simulink model "sgMdl_CAN_FDLoopback"  (R2024b)
settings: Solver=FixedStepAuto  StartTime=0.0  StopTime=inf  RelTol=1e-3  EnableMultiTasking=on
undefined symbols (not defined in the file): CAN, Down, FD, IO602, Pull
libraries: canfdmsglib x7, speedgoatlib_IO602_4 x7, simulink x3, canmsglib x1
Description:
  | CAN - Working with CAN FD
settings Model: ModifiedByFormat=Speedgoat  SimulationMode=external  ExtModeEnableFloating=off  ExtModeTrigDuration=100000  Creator=Speedgoat  LastModifiedBy=Speedgoat
settings SolverCC: ConcurrentTasks=on  AlgebraicLoopSolver=TrustRegion  PositivePriorityOrder=on  AutoInsertRateTranBlk=on  InsertRTBMode=Never (minimum delay)
settings DataIOCC: SaveFormat=StructureWithTime
settings OptimizationCC: BlockReduction=off  OptimizeBlockIOStorage=off  BufferReuse=off  ReuseModelBlockBuffer=off  GlobalBufferReuse=off  ExpressionFolding=off  LocalBlockOutputs=off  OptimizeDataStoreBuffers=off  BusAssignmentInplaceUpdate=off
settings DebuggingCC: InheritedTsInSrcMsg=none  TasksWithSamePriorityMsg=none  ParameterPrecisionLossMsg=none  UnconnectedInputMsg=warning  UnconnectedOutputMsg=warning  UnconnectedLineMsg=warning
settings HardwareCC: ProdBitPerLong=64  ProdLongLongMode=on  ProdHWDeviceType=Intel->x86-64 (Linux 64)
settings ModelReferenceCC: EnableRefExpFcnMdlSchedulingChecks=on
settings SFSimCC: CustomCodeUndefinedFunction=UseInterfaceOnly
settings RTWCC: Description=Speedgoat Real-Time Target Machine  SystemTargetFile=speedgoat.tlc  TemplateMakefile=slrealtime_default_tmf  Toolchain=Simulink Real-Time Toolchain  BuildConfiguration=Faster Runs  TargetLang=C++  GPUComputeCapability=3.5  DLArmComputeVersion=19.05
settings SimulinkRealTimeTargetCC: SubcomponentCodeInterfacePackaging=Reusable function  InstructionSetFMA=off  LogToMDFFile=off  SLRTFileLogMaxRuns=10  UseGCCFastMath=on
settings ConfigComp: CovBoundaryAbsTol=1.0e-5

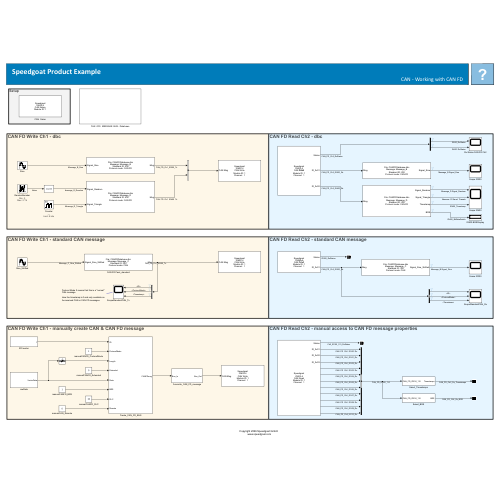
[thumbnail: Simulink's stored preview of the top-level diagram]
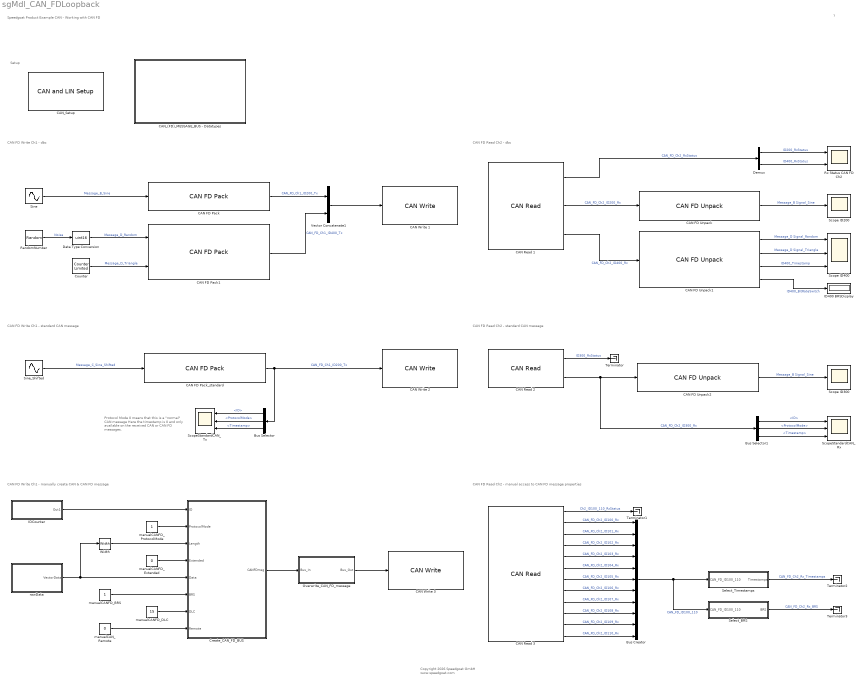
== system sgMdl_CAN_FDLoopback ==
  note: Setup
  note: CAN FD Write Ch1 - dbc
  note: CAN FD Read Ch2 - dbc
  note: CAN FD Write Ch1 - standard CAN message
  note: CAN FD Read Ch2 - standard CAN message
  note: CAN FD Write Ch1 - manually create CAN & CAN FD message
  note: CAN FD Read Ch2 - manual access to CAN FD message properties
  note: Protocol Mode 0 means that this is a "normal" CAN message
      |
      | Here the timestamp is 0 and only available on the received CAN or CAN FD messages.
  note: Speedgoat Product Example
      | CAN - Working with CAN FD
  note: ?
  note: Copyright 2026 Speedgoat GmbH
      |  www.speedgoat.com
  Bus Creator : BusCreator  Inputs=11
  Bus Selector : BusSelector  OutputSignals=ID,ProtocolMode,Timestamp
  Bus Selector1 : BusSelector  OutputSignals=ID,ProtocolMode,Timestamp
  CAN FD Pack : canfdmsglib/CAN FD Pack  CANdbFile=CANFDDatabase.dbc  MsgList=(none)  MsgName=Message_B  ProtocolMode=CAN FD  MsgIDType=Standard (11-bit identifier)  MsgIdentifier=200  CANIDInput=off  MsgLength=8  Remote=off  BRSSwitch=on  ApplyMinMax=off  SignalInfo={'Signal_Sine','0','64','LE','double','Standard','0','1','0','-1.7e+308','1.7e+308'}
      settings: DataFormat=CANdb specified signals
  CAN FD Pack1 : canfdmsglib/CAN FD Pack  CANdbFile=CANFDDatabase.dbc  MsgList=(none)  MsgName=Message_D  ProtocolMode=CAN FD  MsgIDType=Standard (11-bit identifier)  MsgIdentifier=400  CANIDInput=off  MsgLength=3  Remote=off  BRSSwitch=on  ApplyMinMax=off  SignalInfo={'Signal_Random','0','16','LE','unsigned','Standard','0','1','0','0','65535';'Signal_Triangle','16','8','LE','signed','Standard','0','1','0','-128','127'}
      settings: DataFormat=CANdb specified signals
  CAN FD Pack_standard : canfdmsglib/CAN FD Pack  CANdbFile=CANFDDatabase.dbc  MsgList=(none)  MsgName=Message_C  ProtocolMode=CAN  MsgIDType=Standard (11-bit identifier)  MsgIdentifier=300  CANIDInput=off  MsgLength=8  Remote=off  BRSSwitch=off  ApplyMinMax=off  SignalInfo={'Signal_Sine_Shifted','0','64','LE','double','Standard','0','1','0','-1.7e+308','1.7e+308'}
      settings: DataFormat=CANdb specified signals
  CAN FD Unpack : canfdmsglib/CAN FD Unpack  CANdbFile=CANFDDatabase.dbc  MsgList=(none)  MsgName=Message_B  ProtocolMode=CAN FD  MsgIDType=Standard (11-bit identifier)  MsgIdentifier=200  MsgLength=8  SignalInfo={'Signal_Sine','0','64','LE','double','Standard','0','1','0','-1.7e+308','1.7e+308'}  IDPort=off  TimestampPort=off  ErrorPort=off  RemotePort=off  LengthPort=off  StatusPort=off  BRSPort=off  ESIPort=off  DLCPort=off  ApplyMinMax=off
      settings: DataFormat=CANdb specified signals
  CAN FD Unpack1 : canfdmsglib/CAN FD Unpack  CANdbFile=CANFDDatabase.dbc  MsgList=(none)  MsgName=Message_D  ProtocolMode=CAN FD  MsgIDType=Standard (11-bit identifier)  MsgIdentifier=400  MsgLength=3  SignalInfo={'Signal_Random','0','16','LE','unsigned','Standard','0','1','0','0','65535';'Signal_Triangle','16','8','LE','signed','Standard','0','1','0','-128','127'}  IDPort=off  TimestampPort=on  ErrorPort=off  RemotePort=off  LengthPort=off  StatusPort=off  BRSPort=on  ESIPort=off  DLCPort=off  ApplyMinMax=off
      settings: DataFormat=CANdb specified signals
  CAN FD Unpack2 : canfdmsglib/CAN FD Unpack  CANdbFile=CANFDDatabase.dbc  MsgList=(none)  MsgName=Message_C  ProtocolMode=CAN  MsgIDType=Standard (11-bit identifier)  MsgIdentifier=300  MsgLength=8  SignalInfo={'Signal_Sine_Shifted','0','64','LE','double','Standard','0','1','0','-1.7e+308','1.7e+308'}  IDPort=off  TimestampPort=off  ErrorPort=off  RemotePort=off  LengthPort=off  StatusPort=off  BRSPort=off  ESIPort=off  DLCPort=off  ApplyMinMax=off
      settings: DataFormat=CANdb specified signals
  CAN Read 1 : speedgoatlib_IO602_4/CAN Read   moduleType=IO602-4  id=1  channel=2  messageType=CAN (HS)  useBusOut=on  HasMulRead=Specify by IDs  MsgIDlist=[200,400]  isEFF=off  LabelInHex=off  enableInput=off  initValues=[6024 1 -1 1 2 2 0 1 2 0 2 200 400]  ts=-1
      settings: SourceProductName=Simulink Real-Time: Speedgoat I/O Blockset
  CAN Read 2 : speedgoatlib_IO602_4/CAN Read   moduleType=IO602-4  id=1  channel=2  messageType=CAN (HS)  useBusOut=on  HasMulRead=Specify by IDs  MsgIDlist=300  isEFF=off  LabelInHex=off  enableInput=off  initValues=[6024 1 -1 1 2 2 0 1 2 0 1 300]  ts=-1
      settings: SourceProductName=Simulink Real-Time: Speedgoat I/O Blockset
  CAN Read 3 : speedgoatlib_IO602_4/CAN Read   moduleType=IO602-4  id=1  channel=2  messageType=CAN (HS)  useBusOut=on  HasMulRead=Specify by IDs  MsgIDlist=100:110  isEFF=off  LabelInHex=off  enableInput=off  initValues=[6024 1 -1 1 2 2 0 1 2 0 11 100 101 102 103 104 105 106 107 108 109 110]  ts=-1
      settings: SourceProductName=Simulink Real-Time: Speedgoat I/O Blockset
  CAN Write 1 : speedgoatlib_IO602_4/CAN Write   moduleType=IO602-4  id=1  channel=1  messageType=CAN-FD  useBusIn=on  numOfMsg=2  enableInput=off  enableStatusPort=off  ts=-1  initValues=[6024 1 -1 0 2 2 0 2 0 1]
      settings: SourceProductName=Simulink Real-Time: Speedgoat I/O Blockset
  CAN Write 2 : speedgoatlib_IO602_4/CAN Write   moduleType=IO602-4  id=1  channel=1  messageType=CAN-FD  useBusIn=on  numOfMsg=1  enableInput=off  enableStatusPort=off  ts=-1  initValues=[6024 1 -1 0 2 2 0 1 0 1]
      settings: SourceProductName=Simulink Real-Time: Speedgoat I/O Blockset
  CAN Write 3 : speedgoatlib_IO602_4/CAN Write   moduleType=IO602-4  id=1  channel=1  messageType=CAN-FD  useBusIn=on  numOfMsg=1  enableInput=off  enableStatusPort=off  ts=-1  initValues=[6024 1 -1 0 2 2 0 1 0 1]
      settings: SourceProductName=Simulink Real-Time: Speedgoat I/O Blockset
  CAN_(FD)_MESSAGE_BUS - Datatypes : Subsystem
  CAN_Setup : speedgoatlib_IO602_4/CAN and LIN Setup   moduleInitValues="[6024     1     1    -1    -1]"  id=1  moduleType=IO602-4  pciSlot=-1  canChn1=CAN-FD  canChn2=CAN-FD  canChn3=Disabled  canChn4=Disabled  linChn1=Disabled  linChn2=Disabled  canInitStructArray=[]  canTermStructArray=[]  gpioChnx=Disabled  canChn1InitValues="[3   0   2   8  31   8  19   2   2   5   2]"  arbBdrChn1=1.0 MBaud  clockDividerChn1=Enable  arbManBdrChn1=[2,8,31,8]  fdBdrChn1=5.0 MBaud  fdManBdrChn1=[2,2,5,2]  termResistor1=off  canChn2InitValues="[3   0   2   8  31   8  19   2   2   5   2]"  arbBdrChn2=1.0 MBaud  clockDividerChn2=Enable  arbManBdrChn2=[2,8,31,8]  fdBdrChn2=5.0 MBaud  fdManBdrChn2=[2,2,5,2]  termResistor2=off  canChn3InitValues="[1   0   2   8  31   8  19   2   2   5   2]"  arbBdrChn3=1.0 MBaud  clockDividerChn3=Enable  arbManBdrChn3=[2,8,31,8]  fdBdrChn3=5.0 MBaud  fdManBdrChn3=[2,2,5,2]  termResistor3=off  canChn4InitValues="[1   0   2   8  31   8  19   2   2   5   2]"  arbBdrChn4=1.0 MBaud  clockDividerChn4=Enable  arbManBdrChn4=[2,8,31,8]  fdBdrChn4=5.0 MBaud  fdManBdrChn4=[2,2,5,2]  termResistor4=off  linChn1InitValues="[0  9600]"  linBtrChn1=9600  linChn2InitValues="[0  9600]"  linBtrChn2=9600  doInitTermStruct="[0  5  0  0  0]"  parDoChannels=[1 2]  parDoVoltage=5  parDoInitValues=0  parDoReset=1  parNumOfDoS=0  parDiChannels=[3 4]  parDiVoltage=5  parDiPull=Pull-Down
      settings: SourceProductName=Simulink Real-Time: Speedgoat I/O Blockset
  Counter : simulink/Sources/Counter Limited  uplimit=8  tsamp=-1
      settings: AttributesFormatString=|
      | ---
      | Limit: %<uplimit> bits
  Create_CAN_FD_BUS : Subsystem
  Data Type Conversion : DataTypeConversion  OutDataTypeStr=uint16  SaturateOnIntegerOverflow=off  RndMeth=Floor
  Demux : Demux  Outputs=2
  ID400 BRSDisplay : Display
  IDCounter : Subsystem
  Overwrite_CAN_FD_message : Subsystem
  RandomNumber : UniformRandomNumber  Minimum=0  Maximum=2^16  SampleTime=0.01
      settings: AttributesFormatString=|
      | Min: %<Minimum>
      | Max: %<Maximum>
  Rx Status CAN FD Ch2 : Scope  NumInputPorts=2
  Scope ID200 : Scope
  Scope ID300 : Scope
  Scope ID400 : Scope  NumInputPorts=3
  ScopeStandardCAN_Rx : Scope  NumInputPorts=3
  ScopeStandardCAN_Tx : Scope  NumInputPorts=3
  Select_BRS : Subsystem
  Select_Timestamps : Subsystem
  Sine : Sin  Amplitude=255  Frequency=2*pi  SampleTime=0.010
  Sine_Shifted : Sin  Amplitude=255  Bias=pi  Frequency=2*pi  SampleTime=0.010
  Terminator{,1..3} (4 alike) : Terminator
  Vector Concatenate1 : Concatenate
  Width : Width  OutDataTypeMode=All ports same datatype
  manualCANFD_BRS : Constant  OutDataTypeStr=Inherit: Inherit via back propagation  SampleTime=-1
  manualCANFD_DLC : Constant  Value=15  OutDataTypeStr=Inherit: Inherit via back propagation  SampleTime=-1
  manualCANFD_Extended : Constant  Value=0  OutDataTypeStr=Inherit: Inherit via back propagation  SampleTime=-1
  manualCANFD_ProtocolMode : Constant  OutDataTypeStr=Inherit: Inherit via back propagation  SampleTime=-1
  manualCAN_Remote : Constant  Value=0  OutDataTypeStr=Inherit: Inherit via back propagation  SampleTime=-1
  rawData : Subsystem
  wires:
  CAN FD Pack/1 -> Vector Concatenate1/1  "CAN_FD_Ch1_ID200_Tx"
  Vector Concatenate1/1 -> CAN Write 1/1
  Sine/1 -> CAN FD Pack/1  "Message_B_Sine"
  RandomNumber/1 -> Data Type Conversion/1  "Noise"
  Data Type Conversion/1 -> CAN FD Pack1/1  "Message_D_Random"
  Counter/1 -> CAN FD Pack1/2  "Message_D_Triangle"
  CAN FD Pack1/1 -> Vector Concatenate1/2  "CAN_FD_Ch1_ID400_Tx"
  CAN Read 1/1 -> Demux/1  "CAN_FD_Ch2_RxStatus"
  CAN Read 1/2 -> CAN FD Unpack/1  "CAN_FD_Ch2_ID200_Rx"
  CAN Read 1/3 -> CAN FD Unpack1/1  "CAN_FD_Ch2_ID400_Rx"
  CAN FD Unpack/1 -> Scope ID200/1  "Message_B Signal_Sine"
  CAN FD Unpack1/1 -> Scope ID400/1  "Message_D Signal_Random"
  CAN FD Unpack1/2 -> Scope ID400/2  "Message_D Signal_Triangle"
  CAN FD Unpack1/3 -> Scope ID400/3  "ID400_Timestamp"
  CAN FD Unpack1/4 -> ID400 BRSDisplay/1  "ID400_BitRateSwitch"
  Demux/1 -> Rx Status CAN FD Ch2/1  "ID200_RxStatus"
  Demux/2 -> Rx Status CAN FD Ch2/2  "ID400_RxStatus"
  CAN FD Pack_standard/1 -> Bus Selector/1, CAN Write 2/1  "CAN_FD_Ch1_ID200_Tx"
  Sine_Shifted/1 -> CAN FD Pack_standard/1  "Message_C_Sine_Shifted"
  Bus Selector/1 -> ScopeStandardCAN_Tx/1  "<ID>"
  Bus Selector/2 -> ScopeStandardCAN_Tx/2  "<ProtocolMode>"
  Bus Selector/3 -> ScopeStandardCAN_Tx/3  "<Timestamp>"
  CAN Read 2/2 -> Bus Selector1/1, CAN FD Unpack2/1  "CAN_FD_Ch2_ID300_Rx"
  CAN FD Unpack2/1 -> Scope ID300/1  "Message_B Signal_Sine"
  CAN Read 2/1 -> Terminator/1  "ID300_RxStatus"
  IDCounter/1(Out1) -> Create_CAN_FD_BUS/1(ID)
  rawData/1(VectorData) -> Create_CAN_FD_BUS/5(Data), Width/1
  manualCANFD_Extended/1 -> Create_CAN_FD_BUS/4(Extended)
  manualCANFD_DLC/1 -> Create_CAN_FD_BUS/7(DLC)
  Width/1 -> Create_CAN_FD_BUS/3(Length)
  manualCANFD_BRS/1 -> Create_CAN_FD_BUS/6(BRS)
  Create_CAN_FD_BUS/1(CANFDmsg) -> Overwrite_CAN_FD_message/1(Bus_In)
  Overwrite_CAN_FD_message/1(Bus_Out) -> CAN Write 3/1
  CAN Read 3/9 -> Bus Creator/8  "CAN_FD_Ch2_ID107_Rx"
  CAN Read 3/12 -> Bus Creator/11  "CAN_FD_Ch2_ID110_Rx"
  CAN Read 3/8 -> Bus Creator/7  "CAN_FD_Ch2_ID106_Rx"
  CAN Read 3/7 -> Bus Creator/6  "CAN_FD_Ch2_ID105_Rx"
  CAN Read 3/3 -> Bus Creator/2  "CAN_FD_Ch2_ID101_Rx"
  CAN Read 3/4 -> Bus Creator/3  "CAN_FD_Ch2_ID102_Rx"
  CAN Read 3/5 -> Bus Creator/4  "CAN_FD_Ch2_ID103_Rx"
  CAN Read 3/2 -> Bus Creator/1  "CAN_FD_Ch2_ID100_Rx"
  CAN Read 3/1 -> Terminator1/1  "Ch2_ID100_110_RxStatus"
  CAN Read 3/6 -> Bus Creator/5  "CAN_FD_Ch2_ID104_Rx"
  CAN Read 3/11 -> Bus Creator/10  "CAN_FD_Ch2_ID109_Rx"
  CAN Read 3/10 -> Bus Creator/9  "CAN_FD_Ch2_ID108_Rx"
  Bus Selector1/1 -> ScopeStandardCAN_Rx/1  "<ID>"
  Select_BRS/1(BRS) -> Terminator3/1  "CAN_FD_Ch2_Rx_BRS"
  Bus Creator/1 -> Select_Timestamps/1(CAN_FD_ID100_110), Select_BRS/1(CAN_FD_ID100_110)  "CAN_FD_ID100_110"
  Select_Timestamps/1(Timestamps) -> Terminator2/1  "CAN_FD_Ch2_Rx_Timestamps"
  Bus Selector1/3 -> ScopeStandardCAN_Rx/3  "<Timestamp>"
  Bus Selector1/2 -> ScopeStandardCAN_Rx/2  "<ProtocolMode>"
  manualCANFD_ProtocolMode/1 -> Create_CAN_FD_BUS/2(ProtocolMode)
  manualCAN_Remote/1 -> Create_CAN_FD_BUS/8(Remote)

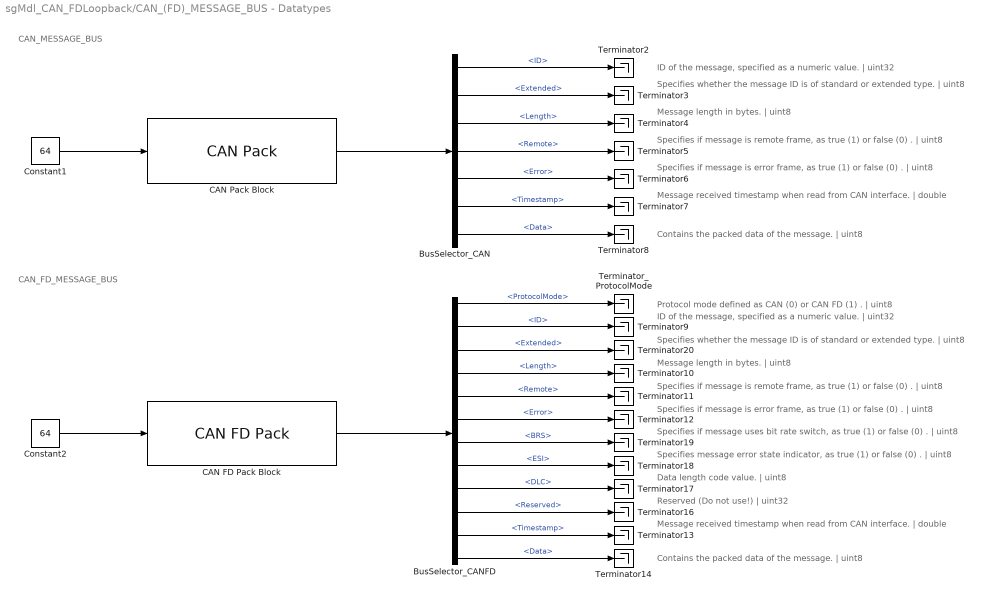
== system sgMdl_CAN_FDLoopback/CAN_(FD)_MESSAGE_BUS - Datatypes ==
  note: CAN_FD_MESSAGE_BUS
  note: Specifies message error state indicator, as true (1) or false (0) . | uint8
  note: ID of the message, specified as a numeric value. | uint32
  note: Contains the packed data of the message. | uint8
  note: Protocol mode defined as CAN (0) or CAN FD (1) . | uint8
  note: Reserved (Do not use!) | uint32
  note: Message received timestamp when read from CAN interface. | double
  note: Specifies if message uses bit rate switch, as true (1) or false (0) . | uint8
  note: Data length code value. | uint8
  note: Specifies whether the message ID is of standard or extended type. | uint8
  note: CAN_MESSAGE_BUS
  note: Specifies if message is error frame, as true (1) or false (0) . | uint8
  note: Message received timestamp when read from CAN interface. | double
  note: Message length in bytes. | uint8
  note: Specifies whether the message ID is of standard or extended type. | uint8
  note: Contains the packed data of the message. | uint8
  note: Message length in bytes. | uint8
  note: Specifies if message is remote frame, as true (1) or false (0) . | uint8
  note: ID of the message, specified as a numeric value. | uint32
  note: Specifies if message is error frame, as true (1) or false (0) . | uint8
  note: Specifies if message is remote frame, as true (1) or false (0) . | uint8
  BusSelector_CAN : BusSelector  OutputSignals=ID,Extended,Length,Remote,Error,Timestamp,Data
  BusSelector_CANFD : BusSelector  OutputSignals=ProtocolMode,ID,Extended,Length,Remote,Error,BRS,ESI,DLC,Reserved,Timestamp,Data
  CAN FD Pack Block : canfdmsglib/CAN FD Pack  MsgList=(none)  MsgName=Msg  ProtocolMode=CAN FD  MsgIDType=Extended (29-bit identifier)  MsgIdentifier=1  CANIDInput=off  MsgLength=16  Remote=off  BRSSwitch=on  ApplyMinMax=off  SignalInfo={}
      settings: DataFormat=raw data
  CAN Pack Block : canmsglib/CAN Pack  MsgList=(none)  MsgName=CAN Msg  MsgIDType=Standard (11-bit identifier)  MsgIdentifier=1  CANIDInput=off  MsgLength=8  Remote=off  ApplyMinMax=off  BusOutput=on  SignalInfo={}
      settings: DataFormat=raw data
  Constant1 : Constant  Value=64  OutDataTypeStr=Inherit: Inherit via back propagation  SampleTime=-1
  Constant2 : Constant  Value=64  OutDataTypeStr=Inherit: Inherit via back propagation  SampleTime=-1
  Terminator{2..14,16..20} (18 alike) : Terminator
  Terminator_ProtocolMode : Terminator
  wires:
  BusSelector_CAN/4 -> Terminator5/1  "<Remote>"
  BusSelector_CANFD/8 -> Terminator18/1  "<ESI>"
  BusSelector_CANFD/7 -> Terminator19/1  "<BRS>"
  BusSelector_CANFD/10 -> Terminator16/1  "<Reserved>"
  Constant2/1 -> CAN FD Pack Block/1
  Constant1/1 -> CAN Pack Block/1
  BusSelector_CANFD/9 -> Terminator17/1  "<DLC>"
  BusSelector_CANFD/1 -> Terminator_ProtocolMode/1  "<ProtocolMode>"
  BusSelector_CANFD/6 -> Terminator12/1  "<Error>"
  BusSelector_CAN/2 -> Terminator3/1  "<Extended>"
  BusSelector_CANFD/5 -> Terminator11/1  "<Remote>"
  BusSelector_CAN/6 -> Terminator7/1  "<Timestamp>"
  BusSelector_CAN/5 -> Terminator6/1  "<Error>"
  BusSelector_CANFD/11 -> Terminator13/1  "<Timestamp>"
  BusSelector_CANFD/4 -> Terminator10/1  "<Length>"
  BusSelector_CAN/1 -> Terminator2/1  "<ID>"
  CAN Pack Block/1 -> BusSelector_CAN/1
  BusSelector_CAN/7 -> Terminator8/1  "<Data>"
  BusSelector_CANFD/2 -> Terminator9/1  "<ID>"
  BusSelector_CANFD/3 -> Terminator20/1  "<Extended>"
  BusSelector_CAN/3 -> Terminator4/1  "<Length>"
  CAN FD Pack Block/1 -> BusSelector_CANFD/1
  BusSelector_CANFD/12 -> Terminator14/1  "<Data>"

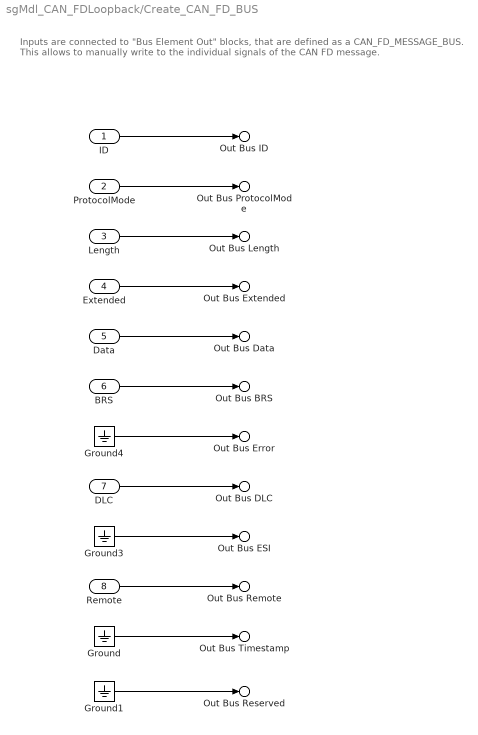
== system sgMdl_CAN_FDLoopback/Create_CAN_FD_BUS ==
  note: Inputs are connected to "Bus Element Out" blocks, that are defined as a CAN_FD_MESSAGE_BUS.
      | This allows to manually write to the individual signals of the CAN FD message.
  ID : Inport
  ProtocolMode : Inport  Port=2
  Length : Inport  Port=3
  Extended : Inport  Port=4
  Data : Inport  Port=5
  BRS : Inport  Port=6
  DLC : Inport  Port=7
  Remote : Inport  Port=8
  Ground{,1,3..4} (4 alike) : Ground
  Out Bus ProtocolMode : Outport  PortName=CANFDmsg  Element=ProtocolMode
  Out Bus Extended : Outport  PortName=CANFDmsg  Element=Extended
  Out Bus Length : Outport  PortName=CANFDmsg  Element=Length
  Out Bus Remote : Outport  PortName=CANFDmsg  Element=Remote
  Out Bus Error : Outport  PortName=CANFDmsg  Element=Error
  Out Bus BRS : Outport  PortName=CANFDmsg  Element=BRS
  Out Bus ESI : Outport  PortName=CANFDmsg  Element=ESI
  Out Bus DLC : Outport  PortName=CANFDmsg  Element=DLC
  Out Bus ID : Outport  PortName=CANFDmsg  Element=ID
  Out Bus Reserved : Outport  PortName=CANFDmsg  Element=Reserved
  Out Bus Timestamp : Outport  PortName=CANFDmsg  Element=Timestamp
  Out Bus Data : Outport  PortName=CANFDmsg  Element=Data
  wires:
  ID/1 -> Out Bus ID/1
  ProtocolMode/1 -> Out Bus ProtocolMode/1
  Length/1 -> Out Bus Length/1
  Extended/1 -> Out Bus Extended/1
  Data/1 -> Out Bus Data/1
  BRS/1 -> Out Bus BRS/1
  Ground4/1 -> Out Bus Error/1
  DLC/1 -> Out Bus DLC/1
  Ground3/1 -> Out Bus ESI/1
  Remote/1 -> Out Bus Remote/1
  Ground/1 -> Out Bus Timestamp/1
  Ground1/1 -> Out Bus Reserved/1

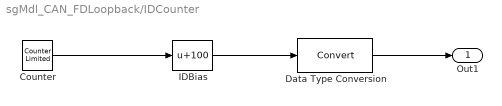
== system sgMdl_CAN_FDLoopback/IDCounter ==
  Counter : simulink/Sources/Counter Limited  uplimit=10  tsamp=-1
      settings: AttributesFormatString=|
      | ---
      | Limit: %<uplimit>
  Data Type Conversion : DataTypeConversion  SaturateOnIntegerOverflow=off  RndMeth=Floor
  IDBias : Bias  Bias=100  SaturateOnIntegerOverflow=off
  Out1 : Outport
  wires:
  IDBias/1 -> Data Type Conversion/1
  Counter/1 -> IDBias/1
  Data Type Conversion/1 -> Out1/1

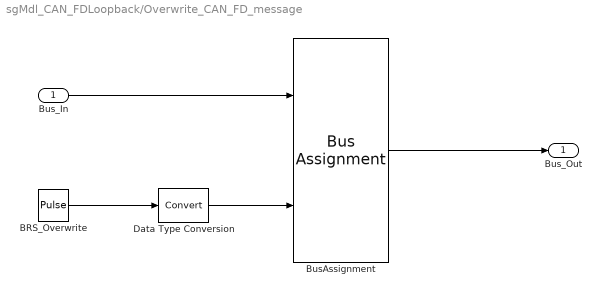
== system sgMdl_CAN_FDLoopback/Overwrite_CAN_FD_message ==
  Bus_In : Inport
  BRS_Overwrite : DiscretePulseGenerator  Period=200  PulseWidth=100  SampleTime=0.01
  BusAssignment : BusAssignment  AssignedSignals=BRS
  Data Type Conversion : DataTypeConversion  SaturateOnIntegerOverflow=off  RndMeth=Floor
  Bus_Out : Outport
  wires:
  BRS_Overwrite/1 -> Data Type Conversion/1
  BusAssignment/1 -> Bus_Out/1
  Bus_In/1 -> BusAssignment/1
  Data Type Conversion/1 -> BusAssignment/2

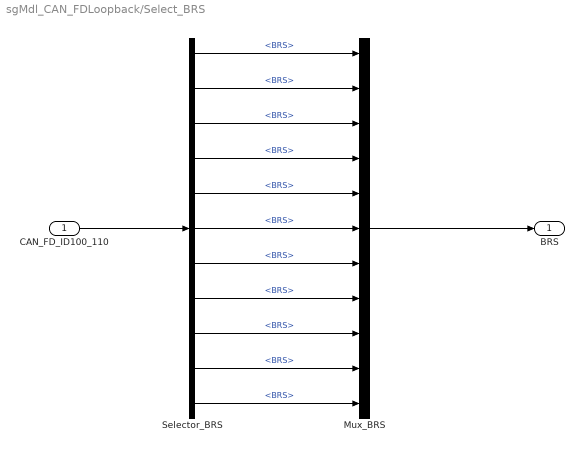
== system sgMdl_CAN_FDLoopback/Select_BRS ==
  CAN_FD_ID100_110 : Inport
  Mux_BRS : Mux  Inputs=11
  Selector_BRS : BusSelector  OutputSignals=CAN_FD_Ch2_ID100_Rx.BRS,CAN_FD_Ch2_ID101_Rx.BRS,CAN_FD_Ch2_ID102_Rx.BRS,CAN_FD_Ch2_ID103_Rx.BRS,CAN_FD_Ch2_ID104_Rx.BRS,CAN_FD_Ch2_ID105_Rx.BRS,CAN_FD_Ch2_ID106_Rx.BRS,CAN_FD_Ch2_ID107_Rx.BRS,CAN_FD_Ch2_ID108_Rx.BRS,CAN_FD_Ch2_ID109_Rx.BRS,CAN_FD_Ch2_ID110_Rx.BRS
  BRS : Outport
  wires:
  CAN_FD_ID100_110/1 -> Selector_BRS/1
  Selector_BRS/10 -> Mux_BRS/10  "<BRS>"
  Selector_BRS/11 -> Mux_BRS/11  "<BRS>"
  Selector_BRS/9 -> Mux_BRS/9  "<BRS>"
  Selector_BRS/8 -> Mux_BRS/8  "<BRS>"
  Selector_BRS/7 -> Mux_BRS/7  "<BRS>"
  Selector_BRS/6 -> Mux_BRS/6  "<BRS>"
  Selector_BRS/5 -> Mux_BRS/5  "<BRS>"
  Selector_BRS/4 -> Mux_BRS/4  "<BRS>"
  Selector_BRS/3 -> Mux_BRS/3  "<BRS>"
  Selector_BRS/2 -> Mux_BRS/2  "<BRS>"
  Selector_BRS/1 -> Mux_BRS/1  "<BRS>"
  Mux_BRS/1 -> BRS/1

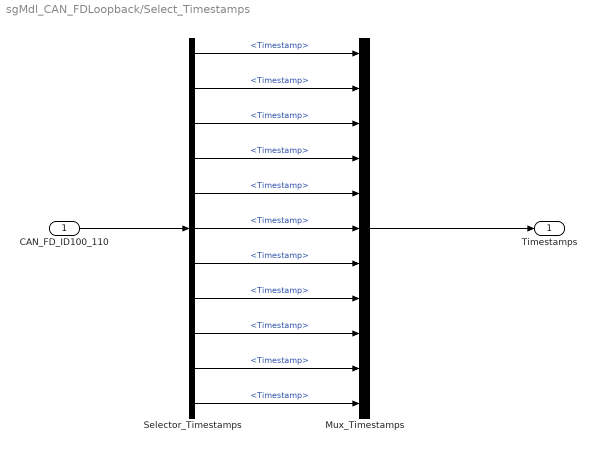
== system sgMdl_CAN_FDLoopback/Select_Timestamps ==
  CAN_FD_ID100_110 : Inport
  Mux_Timestamps : Mux  Inputs=11
  Selector_Timestamps : BusSelector  OutputSignals=CAN_FD_Ch2_ID100_Rx.Timestamp,CAN_FD_Ch2_ID101_Rx.Timestamp,CAN_FD_Ch2_ID102_Rx.Timestamp,CAN_FD_Ch2_ID103_Rx.Timestamp,CAN_FD_Ch2_ID104_Rx.Timestamp,CAN_FD_Ch2_ID105_Rx.Timestamp,CAN_FD_Ch2_ID106_Rx.Timestamp,CAN_FD_Ch2_ID107_Rx.Timestamp,CAN_FD_Ch2_ID108_Rx.Timestamp,CAN_FD_Ch2_ID109_Rx.Timestamp,CAN_FD_Ch2_ID110_Rx.Timestamp
  Timestamps : Outport
  wires:
  Mux_Timestamps/1 -> Timestamps/1
  Selector_Timestamps/1 -> Mux_Timestamps/1  "<Timestamp>"
  Selector_Timestamps/2 -> Mux_Timestamps/2  "<Timestamp>"
  Selector_Timestamps/3 -> Mux_Timestamps/3  "<Timestamp>"
  Selector_Timestamps/4 -> Mux_Timestamps/4  "<Timestamp>"
  Selector_Timestamps/5 -> Mux_Timestamps/5  "<Timestamp>"
  Selector_Timestamps/6 -> Mux_Timestamps/6  "<Timestamp>"
  Selector_Timestamps/7 -> Mux_Timestamps/7  "<Timestamp>"
  Selector_Timestamps/8 -> Mux_Timestamps/8  "<Timestamp>"
  Selector_Timestamps/9 -> Mux_Timestamps/9  "<Timestamp>"
  Selector_Timestamps/11 -> Mux_Timestamps/11  "<Timestamp>"
  Selector_Timestamps/10 -> Mux_Timestamps/10  "<Timestamp>"
  CAN_FD_ID100_110/1 -> Selector_Timestamps/1

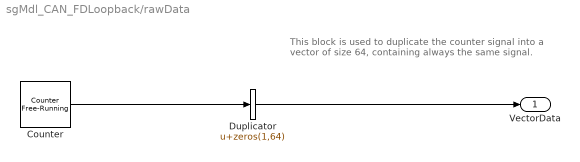
== system sgMdl_CAN_FDLoopback/rawData ==
  note: This block is used to duplicate the counter signal into a vector of size 64, containing always the same signal.
  Counter : simulink/Sources/Counter Free-Running  NumBits=8  tsamp=-1
      settings: AttributesFormatString=|
      | ---
      | Limit: %<NumBits>
  Duplicator : Bias  Bias=zeros(1,64)  SaturateOnIntegerOverflow=off
  VectorData : Outport
  wires:
  Counter/1 -> Duplicator/1
  Duplicator/1 -> VectorData/1
